simulink model "Nonlinear_Simulink"  (R2019b)
settings: Solver=VariableStepAuto  StartTime=0.0  StopTime=6  RelTol=1e-3
libraries: sharedutil x3, vrlib x2, aerolibutil x1
settings Model: Creator=rjgoo  LastModifiedBy=rjgoo
settings DataIOCC: ReturnWorkspaceOutputs=off
settings DebuggingCC: ArithmeticOperatorsInVariantConditions=warning
settings SFSimCC: SimUseLocalCustomCode=off  CustomCodeUndefinedFunction=UseInterfaceOnly
settings RTWCC: RTWUseLocalCustomCode=off

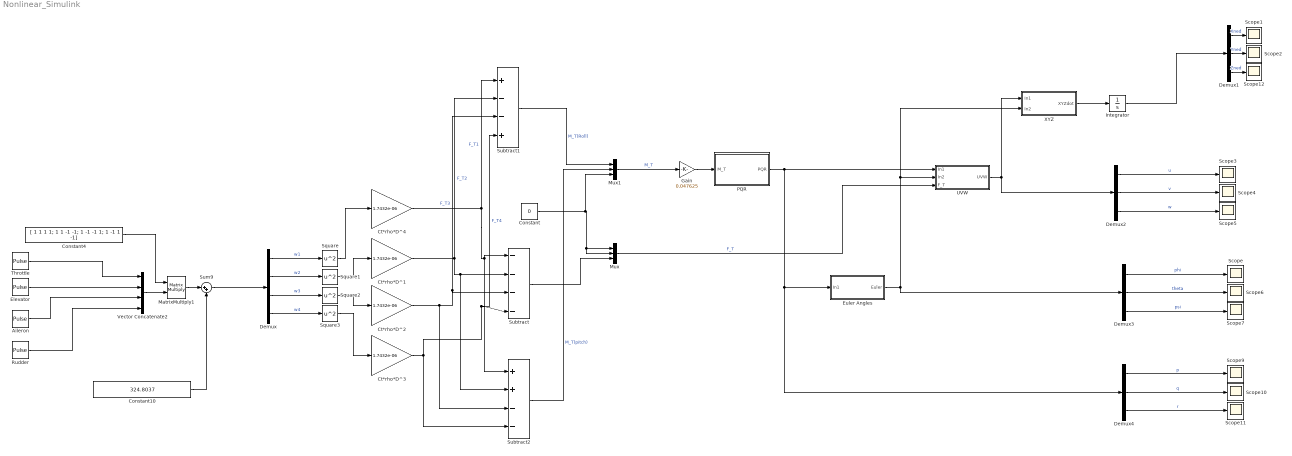
== system Nonlinear_Simulink ==
  Aileron : DiscretePulseGenerator  PulseType=Time based  Amplitude=0.01  Period=8  PulseWidth=50  PhaseDelay=1
  Constant : Constant  Value=0
  Constant10 : Constant  Value=324.8037
  Constant4 : Constant  Value="[ 1 1 1 1; 1 1 -1 -1; 1 -1 -1 1; 1 -1  1 -1]"  VectorParams1D=off
  Ct*rho*D^{1..4} (4 alike) : Gain  Gain=1.7432e-06
  Demux : Demux
  Demux{1..4} (4 alike) : Demux  Outputs=3
  Elevator : DiscretePulseGenerator  PulseType=Time based  Amplitude=0  Period=8  PulseWidth=50  PhaseDelay=1
  Euler Angles : Subsystem
  Gain : Gain  Gain=0.047625
  Integrator : Integrator
  MatrixMultiply1 : Product  Multiplication=Matrix(*)
  Mux : Mux  Inputs=3
  Mux1 : Mux  Inputs=3
  PQR : Subsystem
  Rudder : DiscretePulseGenerator  PulseType=Time based  Amplitude=0  Period=8  PulseWidth=50  PhaseDelay=1
  Scope{,1..7,9..12} (12 alike) : Scope
  Square{,1..3} (4 alike) : Math  Operator=square  SaturateOnIntegerOverflow=on
  Subtract : Sum  Inputs=----
  Subtract1 : Sum  Inputs=+--+
  Subtract2 : Sum  Inputs=++--
  Sum9 : Sum  Inputs=|++
  Throttle : DiscretePulseGenerator  PulseType=Time based  Amplitude=0  Period=8  PulseWidth=50  PhaseDelay=1
  UVW : Subsystem
  Vector Concatenate2 : Concatenate  NumInputs=4
  XYZ : Subsystem
  wires:
  Euler Angles/1(Euler) -> Demux3/1, UVW/2(In2), XYZ/2(In2)
  Constant10/1 -> Sum9/2
  MatrixMultiply1/1 -> Sum9/1
  Constant4/1 -> MatrixMultiply1/1
  Throttle/1 -> Vector Concatenate2/1
  Vector Concatenate2/1 -> MatrixMultiply1/2
  Rudder/1 -> Vector Concatenate2/4
  Aileron/1 -> Vector Concatenate2/3
  Elevator/1 -> Vector Concatenate2/2
  Sum9/1 -> Demux/1
  Demux/1 -> Square/1  "w1"
  Demux/2 -> Square1/1  "w2"
  Demux/3 -> Square2/1  "w3"
  Demux/4 -> Square3/1  "w4"
  Square/1 -> Ct*rho*D^4/1
  Square3/1 -> Ct*rho*D^3/1
  Square2/1 -> Ct*rho*D^2/1
  Square1/1 -> Ct*rho*D^1/1
  Ct*rho*D^4/1 -> Subtract2/1, Subtract/1, Subtract1/1  "F_T1"
  Ct*rho*D^1/1 -> Subtract2/2, Subtract/2, Subtract1/2  "F_T2"
  Ct*rho*D^2/1 -> Subtract2/3, Subtract1/3, Subtract/3  "F_T3"
  Ct*rho*D^3/1 -> Subtract1/4, Subtract/4, Subtract2/4  "F_T4"
  Subtract/1 -> Mux/3
  Mux/1 -> UVW/3(F_T)  "F_T"
  Constant/1 -> Mux1/3, Mux/1, Mux/2
  Subtract1/1 -> Mux1/1  "M_T(Roll)"
  Subtract2/1 -> Mux1/2  "M_T(pitch)"
  Mux1/1 -> Gain/1  "M_T"
  Gain/1 -> PQR/1(M_T)
  UVW/1(UVW) -> XYZ/1(In1), Demux2/1
  Demux2/2 -> Scope4/1  "v"
  Demux2/1 -> Scope3/1  "u"
  Demux2/3 -> Scope5/1  "w"
  Demux3/1 -> Scope/1  "phi"
  Demux3/2 -> Scope6/1  "theta"
  Demux3/3 -> Scope7/1  "psi"
  Demux4/1 -> Scope9/1  "p"
  Demux4/2 -> Scope10/1  "q"
  Demux4/3 -> Scope11/1  "r"
  PQR/1(PQR) -> UVW/1(In1), Demux4/1, Euler Angles/1(In1)
  Demux1/1 -> Scope1/1  "Xned"
  Demux1/3 -> Scope12/1  "Zned"
  Demux1/2 -> Scope2/1  "Yned"
  XYZ/1(XYZdot) -> Integrator/1
  Integrator/1 -> Demux1/1

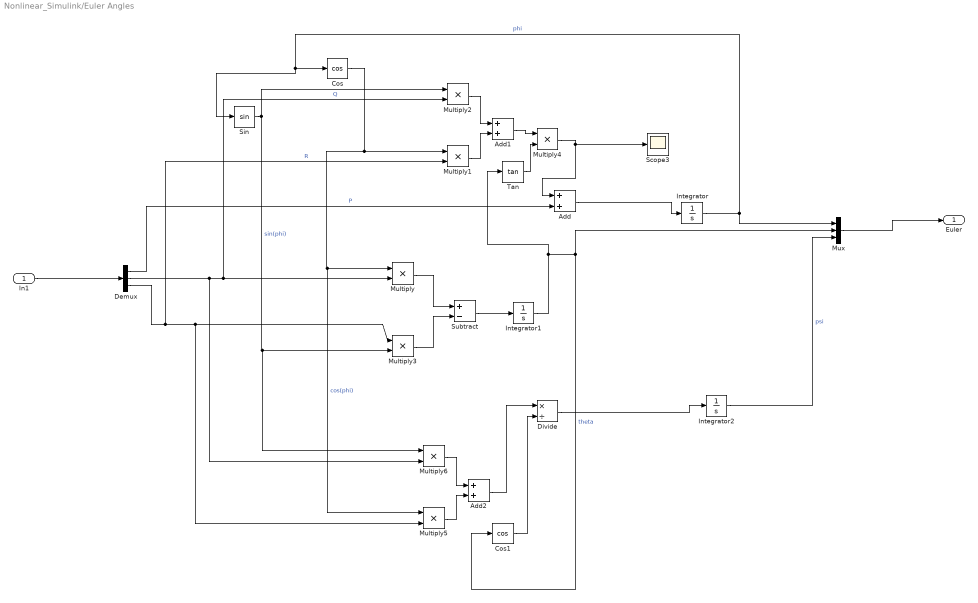
== system Nonlinear_Simulink/Euler Angles ==
  In1 : Inport
  Add : Sum
  Add1 : Sum
  Add2 : Sum
  Cos : Trigonometry  Operator=cos
  Cos1 : Trigonometry  Operator=cos
  Demux : Demux  Outputs=3
  Divide : Product  Inputs=*/
  Integrator : Integrator
  Integrator1 : Integrator
  Integrator2 : Integrator
  Multiply{,1..6} (7 alike) : Product
  Mux : Mux  Inputs=3
  Scope3 : Scope
  Sin : Trigonometry
  Subtract : Sum  Inputs=+-
  Tan : Trigonometry  Operator=tan
  Euler : Outport  VectorParamsAs1DForOutWhenUnconnected=off
  wires:
  In1/1 -> Demux/1
  Integrator/1 -> Cos/1, Sin/1, Mux/1  "phi"
  Integrator1/1 -> Tan/1, Cos1/1, Mux/2  "theta"
  Integrator2/1 -> Mux/3  "psi"
  Mux/1 -> Euler/1
  Multiply/1 -> Subtract/1
  Multiply3/1 -> Subtract/2
  Subtract/1 -> Integrator1/1
  Multiply2/1 -> Add1/1
  Multiply1/1 -> Add1/2
  Tan/1 -> Multiply4/2
  Add1/1 -> Multiply4/1
  Demux/3 -> Multiply1/2, Multiply5/2, Multiply3/1  "R"
  Sin/1 -> Multiply6/1, Multiply3/2, Multiply2/1  "sin(phi)"
  Cos/1 -> Multiply5/1, Multiply/1, Multiply1/1  "cos(phi)"
  Demux/2 -> Multiply6/2, Multiply2/2, Multiply/2  "Q"
  Multiply5/1 -> Add2/2
  Multiply6/1 -> Add2/1
  Add2/1 -> Divide/1
  Cos1/1 -> Divide/2
  Divide/1 -> Integrator2/1
  Demux/1 -> Add/2  "P"
  Multiply4/1 -> Add/1, Scope3/1
  Add/1 -> Integrator/1

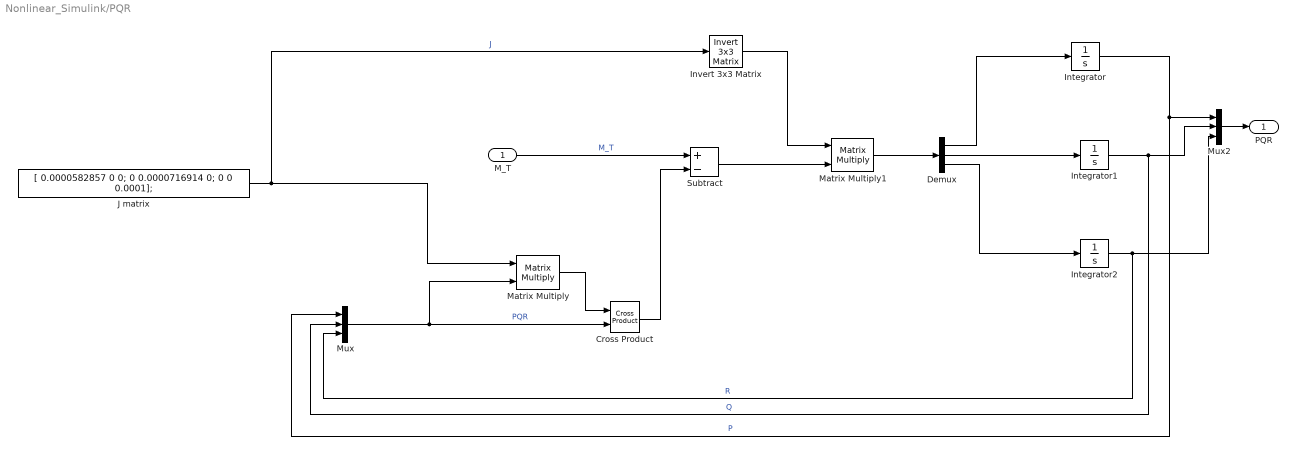
== system Nonlinear_Simulink/PQR ==
  M_T : Inport
  Cross Product : vrlib/Utilities/Cross Product
      settings: SourceProductName=Simulink
  Demux : Demux  Outputs=3
  Integrator : Integrator
  Integrator1 : Integrator
  Integrator2 : Integrator
  Invert 3x3 Matrix : aerolibutil/Invert  3x3 Matrix
  J matrix : Constant  Value=[ 0.0000582857 0 0; 0 0.0000716914 0; 0 0 0.0001];
  Matrix Multiply : Product  Multiplication=Matrix(*)
  Matrix Multiply1 : Product  Multiplication=Matrix(*)
  Mux : Mux  Inputs=3
  Mux2 : Mux  Inputs=3
  Subtract : Sum  Inputs=+-
  PQR : Outport  VectorParamsAs1DForOutWhenUnconnected=off
  wires:
  Integrator/1 -> Mux2/1, Mux/1  "P"
  Integrator1/1 -> Mux/2, Mux2/2  "Q"
  Integrator2/1 -> Mux/3, Mux2/3  "R"
  J matrix/1 -> Invert 3x3 Matrix/1, Matrix Multiply/1  "J"
  M_T/1 -> Subtract/1  "M_T"
  Mux/1 -> Cross Product/2, Matrix Multiply/2  "PQR"
  Matrix Multiply/1 -> Cross Product/1
  Cross Product/1 -> Subtract/2
  Invert 3x3 Matrix/1 -> Matrix Multiply1/1
  Subtract/1 -> Matrix Multiply1/2
  Matrix Multiply1/1 -> Demux/1
  Demux/1 -> Integrator/1
  Demux/2 -> Integrator1/1
  Demux/3 -> Integrator2/1
  Mux2/1 -> PQR/1

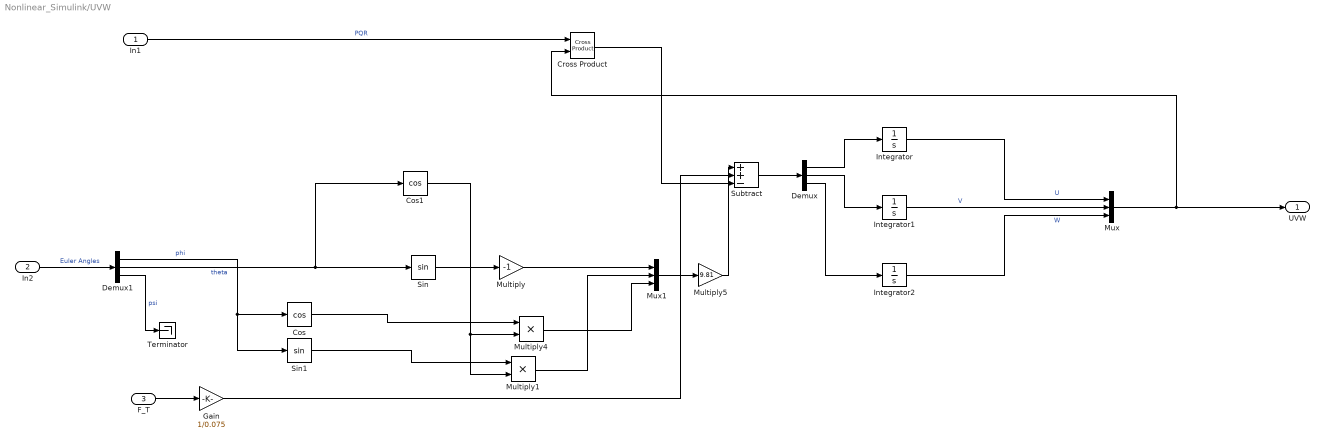
== system Nonlinear_Simulink/UVW ==
  In1 : Inport
  In2 : Inport  Port=2
  F_T : Inport  Port=3
  Cos : Trigonometry  Operator=cos
  Cos1 : Trigonometry  Operator=cos
  Cross Product : vrlib/Utilities/Cross Product
      settings: SourceProductName=Simulink
  Demux : Demux  Outputs=3
  Demux1 : Demux  Outputs=3
  Gain : Gain  Gain=1/0.075
  Integrator : Integrator
  Integrator1 : Integrator
  Integrator2 : Integrator
  Multiply : Gain  Gain=-1
  Multiply1 : Product
  Multiply4 : Product
  Multiply5 : Gain  Gain=9.81
  Mux : Mux  Inputs=3
  Mux1 : Mux  Inputs=3
  Sin : Trigonometry
  Sin1 : Trigonometry
  Subtract : Sum  Inputs=++-
  Terminator : Terminator
  UVW : Outport  VectorParamsAs1DForOutWhenUnconnected=off
  wires:
  In1/1 -> Cross Product/1  "PQR"
  In2/1 -> Demux1/1  "Euler Angles"
  Integrator/1 -> Mux/1  "U"
  Integrator1/1 -> Mux/2  "V"
  Integrator2/1 -> Mux/3  "W"
  Demux1/1 -> Sin1/1, Cos/1  "phi"
  Demux1/2 -> Cos1/1, Sin/1  "theta"
  Demux1/3 -> Terminator/1  "psi"
  Mux/1 -> Cross Product/2, UVW/1
  F_T/1 -> Gain/1
  Demux/3 -> Integrator2/1
  Sin/1 -> Multiply/1
  Multiply/1 -> Mux1/1
  Cos1/1 -> Multiply1/2, Multiply4/2
  Sin1/1 -> Multiply1/1
  Multiply1/1 -> Mux1/2
  Cos/1 -> Multiply4/1
  Multiply4/1 -> Mux1/3
  Mux1/1 -> Multiply5/1
  Multiply5/1 -> Subtract/1
  Gain/1 -> Subtract/2
  Cross Product/1 -> Subtract/3
  Subtract/1 -> Demux/1
  Demux/1 -> Integrator/1
  Demux/2 -> Integrator1/1

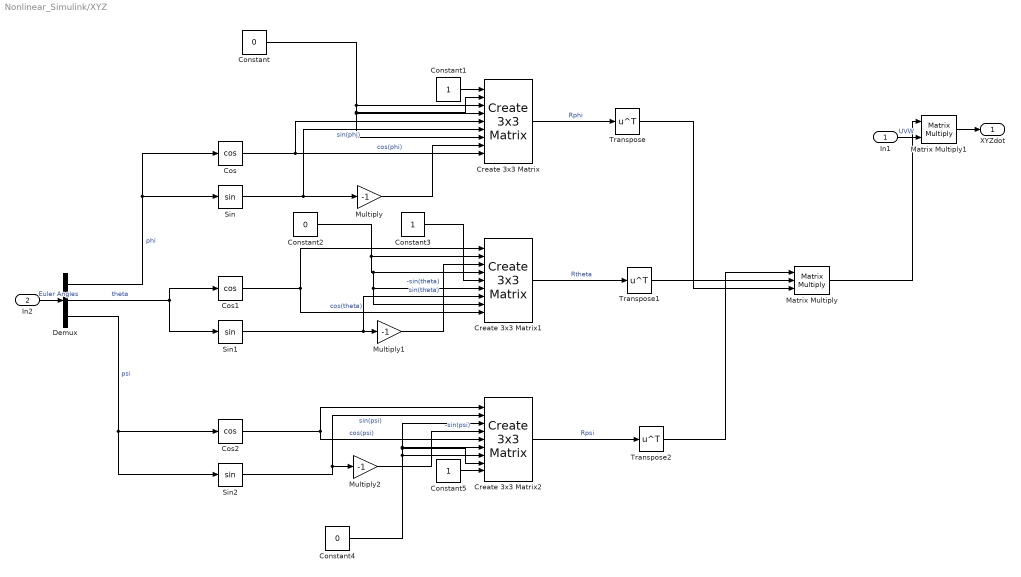
== system Nonlinear_Simulink/XYZ ==
  In1 : Inport
  In2 : Inport  Port=2
  Constant : Constant  Value=0
  Constant1 : Constant
  Constant2 : Constant  Value=0
  Constant3 : Constant
  Constant4 : Constant  Value=0
  Constant5 : Constant
  Cos : Trigonometry  Operator=cos
  Cos1 : Trigonometry  Operator=cos
  Cos2 : Trigonometry  Operator=cos
  Create 3x3 Matrix : sharedutil/Create 3x3 Matrix  aMode=aMode
  Create 3x3 Matrix1 : sharedutil/Create 3x3 Matrix  aMode=aMode
  Create 3x3 Matrix2 : sharedutil/Create 3x3 Matrix  aMode=aMode
  Demux : Demux  Outputs=3
  Matrix Multiply : Product  Inputs=3  Multiplication=Matrix(*)
  Matrix Multiply1 : Product  Multiplication=Matrix(*)
  Multiply : Gain  Gain=-1
  Multiply1 : Gain  Gain=-1
  Multiply2 : Gain  Gain=-1
  Sin : Trigonometry
  Sin1 : Trigonometry
  Sin2 : Trigonometry
  Transpose : Math  Operator=transpose  SignedPower=off  SaturateOnIntegerOverflow=on
  Transpose1 : Math  Operator=transpose  SignedPower=off  SaturateOnIntegerOverflow=on
  Transpose2 : Math  Operator=transpose  SignedPower=off  SaturateOnIntegerOverflow=on
  XYZdot : Outport  VectorParamsAs1DForOutWhenUnconnected=off
  wires:
  In1/1 -> Matrix Multiply1/2  "UVW"
  In2/1 -> Demux/1  "Euler Angles"
  Demux/1 -> Cos/1, Sin/1  "phi"
  Demux/2 -> Sin1/1, Cos1/1  "theta"
  Demux/3 -> Sin2/1, Cos2/1  "psi"
  Create 3x3 Matrix/1 -> Transpose/1  "Rphi"
  Create 3x3 Matrix1/1 -> Transpose1/1  "Rtheta"
  Create 3x3 Matrix2/1 -> Transpose2/1  "Rpsi"
  Constant1/1 -> Create 3x3 Matrix/1
  Constant/1 -> Create 3x3 Matrix/2, Create 3x3 Matrix/7, Create 3x3 Matrix/4, Create 3x3 Matrix/3
  Cos/1 -> Create 3x3 Matrix/5, Create 3x3 Matrix/9  "cos(phi)"
  Sin/1 -> Create 3x3 Matrix/6, Multiply/1  "sin(phi)"
  Multiply/1 -> Create 3x3 Matrix/8
  Cos1/1 -> Create 3x3 Matrix1/1, Create 3x3 Matrix1/9  "cos(theta)"
  Constant2/1 -> Create 3x3 Matrix1/8, Create 3x3 Matrix1/6, Create 3x3 Matrix1/4, Create 3x3 Matrix1/2
  Sin1/1 -> Create 3x3 Matrix1/7, Multiply1/1  "sin(theta)"
  Multiply1/1 -> Create 3x3 Matrix1/3  "-sin(theta)"
  Constant3/1 -> Create 3x3 Matrix1/5
  Cos2/1 -> Create 3x3 Matrix2/1, Create 3x3 Matrix2/5  "cos(psi)"
  Sin2/1 -> Multiply2/1, Create 3x3 Matrix2/2  "sin(psi)"
  Constant4/1 -> Create 3x3 Matrix2/8, Create 3x3 Matrix2/3, Create 3x3 Matrix2/6, Create 3x3 Matrix2/7
  Multiply2/1 -> Create 3x3 Matrix2/4  "-sin(psi)"
  Constant5/1 -> Create 3x3 Matrix2/9
  Transpose2/1 -> Matrix Multiply/1
  Transpose1/1 -> Matrix Multiply/2
  Transpose/1 -> Matrix Multiply/3
  Matrix Multiply/1 -> Matrix Multiply1/1
  Matrix Multiply1/1 -> XYZdot/1
